simulink model "gm_parallel_prediction_and_cost_function_6phase"  (R2022a)
settings: Solver=FixedStepDiscrete  StartTime=0.0  StopTime=10.0  RelTol=1e-3
undefined symbols (not defined in the file or in its folder): f_c, L_d, L_q, L_x, L_y, p, psi_pm, R_ph
libraries: hdlmdlgenlib x2
(part 1 of 8)
settings Model: Creator=Andre Merx  LastModifiedBy=Andre Merx
settings SolverCC: AlgebraicLoopSolver=TrustRegion
settings DataIOCC: LimitDataPoints=on  SaveOutput=off  SaveTime=off
settings OptimizationCC: BlockReduction=off  ConditionallyExecuteInputs=off  DefaultParameterBehavior=Inlined  LifeSpan=inf
settings DebuggingCC: AlgebraicLoopMsg=error  InheritedTsInSrcMsg=none  SingleTaskRateTransMsg=error  UnconnectedInputMsg=warning  UnconnectedOutputMsg=warning  UnconnectedLineMsg=warning  AllowSymbolicDim=off  StrictBusMsg=ErrorOnBusTreatedAsVector  SFUnexpectedBacktrackingDiag=warning  SFNoUnconditionalDefaultTransitionDiag=warning  SFExecutionAtInitializationDiag=none  SFMachineParentedDataDiag=warning  ArithmeticOperatorsInVariantConditions=warning
settings HardwareCC: ProdBitPerPointer=32  ProdBitPerSizeT=32  ProdBitPerPtrDiffT=32  ProdLargestAtomicFloat=None  ProdIntDivRoundTo=Undefined  ProdEndianess=Unspecified  ProdWordSize=32  ProdHWDeviceType=ASIC/FPGA->ASIC/FPGA  ProdEqTarget=off
settings SFSimCC: SimUseLocalCustomCode=off  CustomCodeUndefinedFunction=UseInterfaceOnly
settings RTWCC: RTWUseLocalCustomCode=off
settings CodeAppCC: StateflowObjectComments=on
settings GRTTargetCC: TargetLangStandard=C89/C90 (ANSI)
settings ConfigComp: CovScope=ReferencedModels  CovMetricSettings=dw  CovSaveCumulativeToWorkspaceVar=on  CovSaveSingleToWorkspaceVar=on  CovExternalEMLEnable=off  CovSFcnEnable=off

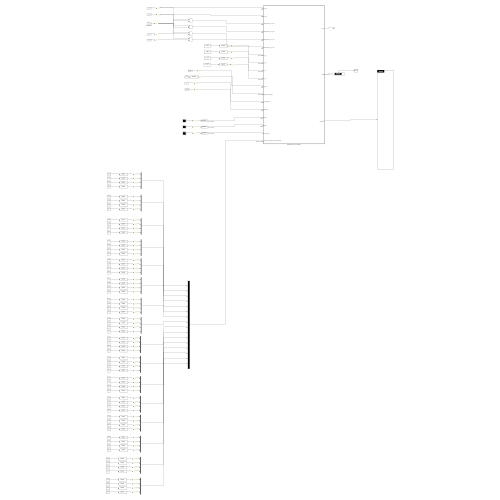
[thumbnail: Simulink's stored preview of the top-level diagram]
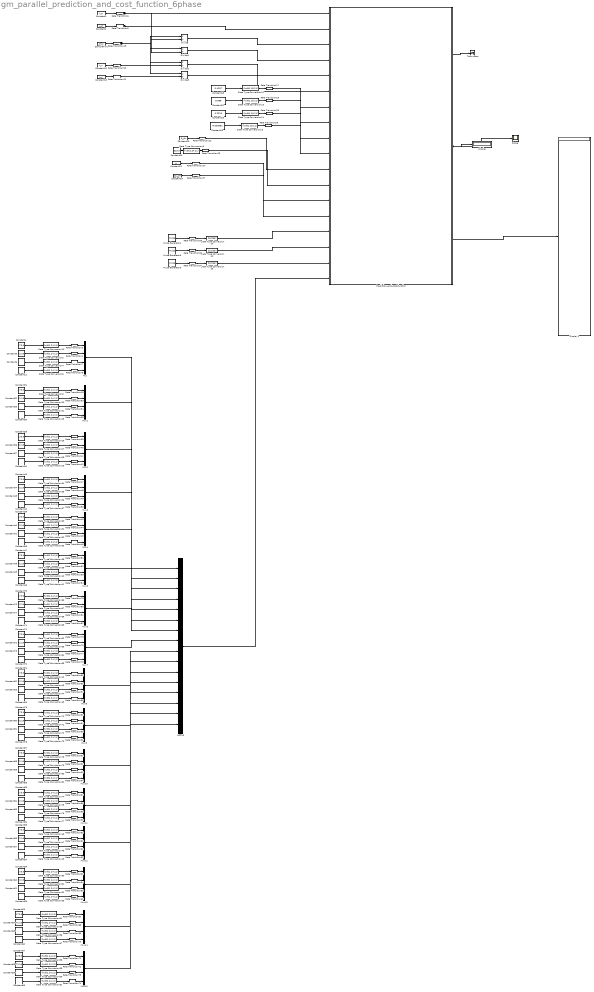
== system gm_parallel_prediction_and_cost_function_6phase ==
  Constant1 : Constant  Value=L_d  OutDataTypeStr=single  SampleTime=-1
  Constant{11,30,34,38,42,46,50,54,58,62,66,70,74,78,82,86} (16 alike) : Constant  Value=-163.1
  Constant12 : Constant  Value=L_x  OutDataTypeStr=single  SampleTime=-1
  Constant13 : Constant  Value=L_y  OutDataTypeStr=single  SampleTime=-1
  Constant18 : Constant  Value=0.4297
  Constant19 : Constant  Value=R_ph  OutDataTypeStr=single  SampleTime=-1
  Constant2 : Constant  Value=L_q  OutDataTypeStr=single  SampleTime=-1
  Constant20 : Constant  Value=313.3
  Constant21 : Constant  Value=p  OutDataTypeStr=single  SampleTime=-1
  Constant22 : Constant  Value=9.988
  Constant23 : Constant  Value=0.2219
  Constant24 : Constant  Value=psi_pm  OutDataTypeStr=single  SampleTime=-1
  Constant25 : Constant  Value=-0.003051
  Constant{4,31,35,39,43,47,51,55,59,63,67,71,75,79,83,87} (16 alike) : Constant  Value=173.9
  Constant{5,32,36,40,44,48,52,56,60,64,68,72,76,80,84,88} (16 alike) : Constant  Value=72.19
  Constant{6,33,37,41,45,49,53,57,61,65,69,73,77,81,85,89} (16 alike) : Constant  Value=-94.17
  Data Type Conversion{2..6,10,20..21,25..81} (65 alike) : DataTypeConversion  OutDataTypeStr=fixdt(1,24,11)  SaturateOnIntegerOverflow=off  RndMeth=Floor
  Data Type Conversion{12..15} (4 alike) : DataTypeConversion  OutDataTypeStr=fixdt(1,18,11)  SaturateOnIntegerOverflow=off  RndMeth=Floor
  Data Type Conversion22 : DataTypeConversion  OutDataTypeStr=boolean  SaturateOnIntegerOverflow=off  RndMeth=Floor
  Data Type Conversion23 : DataTypeConversion  OutDataTypeStr=boolean  SaturateOnIntegerOverflow=off  RndMeth=Floor
  Data Type Conversion24 : DataTypeConversion  OutDataTypeStr=boolean  SaturateOnIntegerOverflow=off  RndMeth=Floor
  Display : Display
  Display1 : Display
  Divide{,1..3} (4 alike) : Product  Inputs=*/  RndMeth=Zero  SaturateOnIntegerOverflow=on
  Mux{,1..15} (16 alike) : Mux
  Mux16 : Mux  Inputs=16
  Prediction_and_cost_function : Subsystem  TreatAsAtomicUnit=on
  Pulse Generator4 : DiscretePulseGenerator  PulseType=Time based  Period=1/f_c
  Pulse Generator5 : DiscretePulseGenerator  PulseType=Time based  Period=1/f_c
  Pulse Generator6 : DiscretePulseGenerator  PulseType=Time based  Period=1/f_c
  Rate Transition{3..8,17..28,33..94} (80 alike) : RateTransition  OutPortSampleTime=Rt
  SampleTime : Constant  Value=1/f_c  OutDataTypeStr=single  SampleTime=-1
  Scope : Scope
  Terminator : Terminator
  wires:
  Prediction_and_cost_function/3(Prediction) -> Display1/1
  Prediction_and_cost_function/1(done) -> Terminator/1
  Prediction_and_cost_function/2(Index) -> Display/1, Scope/1
  Mux16/1 -> Prediction_and_cost_function/18(dqxy_phase_voltage_per_switching_state)
  Mux15/1 -> Mux16/16
  Mux14/1 -> Mux16/15
  Mux13/1 -> Mux16/14
  Mux12/1 -> Mux16/13
  Mux11/1 -> Mux16/12
  Mux10/1 -> Mux16/11
  Mux9/1 -> Mux16/10
  Mux8/1 -> Mux16/9
  Mux7/1 -> Mux16/8
  Mux6/1 -> Mux16/7
  Mux5/1 -> Mux16/6
  Mux4/1 -> Mux16/5
  Mux3/1 -> Mux16/4
  Mux2/1 -> Mux16/3
  Mux1/1 -> Mux16/2
  Mux/1 -> Mux16/1
  Rate Transition74/1 -> Mux15/4
  Rate Transition73/1 -> Mux15/3
  Rate Transition72/1 -> Mux15/2
  Rate Transition71/1 -> Mux15/1
  Rate Transition70/1 -> Mux14/4
  Rate Transition69/1 -> Mux14/3
  Rate Transition68/1 -> Mux14/2
  Rate Transition67/1 -> Mux14/1
  Rate Transition66/1 -> Mux13/4
  Rate Transition65/1 -> Mux13/3
  Rate Transition64/1 -> Mux13/2
  Rate Transition63/1 -> Mux13/1
  Rate Transition62/1 -> Mux12/4
  Rate Transition61/1 -> Mux12/3
  Rate Transition60/1 -> Mux12/2
  Rate Transition59/1 -> Mux12/1
  Rate Transition90/1 -> Mux11/4
  Rate Transition89/1 -> Mux11/3
  Rate Transition88/1 -> Mux11/2
  Rate Transition87/1 -> Mux11/1
  Rate Transition94/1 -> Mux10/4
  Rate Transition93/1 -> Mux10/3
  Rate Transition92/1 -> Mux10/2
  Rate Transition91/1 -> Mux10/1
  Rate Transition86/1 -> Mux9/4
  Rate Transition85/1 -> Mux9/3
  Rate Transition84/1 -> Mux9/2
  Rate Transition83/1 -> Mux9/1
  Rate Transition57/1 -> Mux8/3
  Rate Transition58/1 -> Mux8/4
  Rate Transition56/1 -> Mux8/2
  Rate Transition55/1 -> Mux8/1
  Rate Transition77/1 -> Mux7/3
  Rate Transition78/1 -> Mux7/4
  Rate Transition76/1 -> Mux7/2
  Rate Transition75/1 -> Mux7/1
  Rate Transition82/1 -> Mux6/4
  Rate Transition81/1 -> Mux6/3
  Rate Transition80/1 -> Mux6/2
  Rate Transition79/1 -> Mux6/1
  Rate Transition54/1 -> Mux5/4
  Rate Transition53/1 -> Mux5/3
  Rate Transition52/1 -> Mux5/2
  Rate Transition51/1 -> Mux5/1
  Rate Transition46/1 -> Mux4/4
  Rate Transition45/1 -> Mux4/3
  Rate Transition44/1 -> Mux4/2
  Rate Transition43/1 -> Mux4/1
  Rate Transition50/1 -> Mux3/4
  Rate Transition49/1 -> Mux3/3
  Rate Transition48/1 -> Mux3/2
  Rate Transition47/1 -> Mux3/1
  Rate Transition42/1 -> Mux2/4
  Rate Transition41/1 -> Mux2/3
  Rate Transition40/1 -> Mux2/2
  Rate Transition39/1 -> Mux2/1
  Rate Transition38/1 -> Mux1/4
  Rate Transition34/1 -> Mux1/3
  Rate Transition33/1 -> Mux1/2
  Rate Transition18/1 -> Mux1/1
  Rate Transition8/1 -> Mux/4
  Rate Transition7/1 -> Mux/3
  Rate Transition4/1 -> Mux/2
  Rate Transition3/1 -> Mux/1
  Data Type Conversion58/1 -> Rate Transition71/1
  Data Type Conversion59/1 -> Rate Transition72/1
  Data Type Conversion60/1 -> Rate Transition73/1
  Constant69/1 -> Data Type Conversion60/1
  Constant66/1 -> Data Type Conversion61/1
  Constant67/1 -> Data Type Conversion58/1
  Constant68/1 -> Data Type Conversion59/1
  Data Type Conversion61/1 -> Rate Transition74/1
  Data Type Conversion54/1 -> Rate Transition67/1
  Data Type Conversion55/1 -> Rate Transition68/1
  Data Type Conversion56/1 -> Rate Transition69/1
  Constant65/1 -> Data Type Conversion56/1
  Constant62/1 -> Data Type Conversion57/1
  Constant63/1 -> Data Type Conversion54/1
  Constant64/1 -> Data Type Conversion55/1
  Data Type Conversion57/1 -> Rate Transition70/1
  Data Type Conversion50/1 -> Rate Transition63/1
  Data Type Conversion51/1 -> Rate Transition64/1
  Data Type Conversion52/1 -> Rate Transition65/1
  Constant61/1 -> Data Type Conversion52/1
  Constant58/1 -> Data Type Conversion53/1
  Constant59/1 -> Data Type Conversion50/1
  Constant60/1 -> Data Type Conversion51/1
  Data Type Conversion53/1 -> Rate Transition66/1
  Data Type Conversion78/1 -> Rate Transition91/1
  Data Type Conversion79/1 -> Rate Transition92/1
  Data Type Conversion80/1 -> Rate Transition93/1
  Constant89/1 -> Data Type Conversion80/1
  Constant86/1 -> Data Type Conversion81/1
  Constant87/1 -> Data Type Conversion78/1
  Constant88/1 -> Data Type Conversion79/1
  Data Type Conversion81/1 -> Rate Transition94/1
  Data Type Conversion74/1 -> Rate Transition87/1
  Data Type Conversion75/1 -> Rate Transition88/1
  Data Type Conversion76/1 -> Rate Transition89/1
  Constant85/1 -> Data Type Conversion76/1
  Constant82/1 -> Data Type Conversion77/1
  Constant83/1 -> Data Type Conversion74/1
  Constant84/1 -> Data Type Conversion75/1
  Data Type Conversion77/1 -> Rate Transition90/1
  Data Type Conversion70/1 -> Rate Transition83/1
  Data Type Conversion71/1 -> Rate Transition84/1
  Data Type Conversion72/1 -> Rate Transition85/1
  Constant81/1 -> Data Type Conversion72/1
  Constant78/1 -> Data Type Conversion73/1
  Constant79/1 -> Data Type Conversion70/1
  Constant80/1 -> Data Type Conversion71/1
  Data Type Conversion73/1 -> Rate Transition86/1
  Data Type Conversion66/1 -> Rate Transition79/1
  Data Type Conversion67/1 -> Rate Transition80/1
  Data Type Conversion68/1 -> Rate Transition81/1
  Constant77/1 -> Data Type Conversion68/1
  Constant74/1 -> Data Type Conversion69/1
  Constant75/1 -> Data Type Conversion66/1
  Constant76/1 -> Data Type Conversion67/1
  Data Type Conversion69/1 -> Rate Transition82/1
  Data Type Conversion62/1 -> Rate Transition75/1
  Data Type Conversion63/1 -> Rate Transition76/1
  Data Type Conversion64/1 -> Rate Transition77/1
  Constant73/1 -> Data Type Conversion64/1
  Constant70/1 -> Data Type Conversion65/1
  Constant71/1 -> Data Type Conversion62/1
  Constant72/1 -> Data Type Conversion63/1
  Data Type Conversion65/1 -> Rate Transition78/1
  Data Type Conversion46/1 -> Rate Transition59/1
  Data Type Conversion47/1 -> Rate Transition60/1
  Data Type Conversion48/1 -> Rate Transition61/1
  Constant57/1 -> Data Type Conversion48/1
  Constant54/1 -> Data Type Conversion49/1
  Constant55/1 -> Data Type Conversion46/1
  Constant56/1 -> Data Type Conversion47/1
  Data Type Conversion49/1 -> Rate Transition62/1
  Data Type Conversion42/1 -> Rate Transition55/1
  Data Type Conversion43/1 -> Rate Transition56/1
  Data Type Conversion44/1 -> Rate Transition57/1
  Constant53/1 -> Data Type Conversion44/1
  Constant50/1 -> Data Type Conversion45/1
  Constant51/1 -> Data Type Conversion42/1
  Constant52/1 -> Data Type Conversion43/1
  Data Type Conversion45/1 -> Rate Transition58/1
  Data Type Conversion38/1 -> Rate Transition51/1
  Data Type Conversion39/1 -> Rate Transition52/1
  Data Type Conversion40/1 -> Rate Transition53/1
  Constant49/1 -> Data Type Conversion40/1
  Constant46/1 -> Data Type Conversion41/1
  Constant47/1 -> Data Type Conversion38/1
  Constant48/1 -> Data Type Conversion39/1
  Data Type Conversion41/1 -> Rate Transition54/1
  Data Type Conversion34/1 -> Rate Transition47/1
  Data Type Conversion35/1 -> Rate Transition48/1
  Data Type Conversion36/1 -> Rate Transition49/1
  Constant45/1 -> Data Type Conversion36/1
  Constant42/1 -> Data Type Conversion37/1
  Constant43/1 -> Data Type Conversion34/1
  Constant44/1 -> Data Type Conversion35/1
  Data Type Conversion37/1 -> Rate Transition50/1
  Data Type Conversion30/1 -> Rate Transition43/1
  Data Type Conversion31/1 -> Rate Transition44/1
  Data Type Conversion32/1 -> Rate Transition45/1
  Constant41/1 -> Data Type Conversion32/1
  Constant38/1 -> Data Type Conversion33/1
  Constant39/1 -> Data Type Conversion30/1
  Constant40/1 -> Data Type Conversion31/1
  Data Type Conversion33/1 -> Rate Transition46/1
  Data Type Conversion26/1 -> Rate Transition39/1
  Data Type Conversion27/1 -> Rate Transition40/1
  Data Type Conversion28/1 -> Rate Transition41/1
  Constant37/1 -> Data Type Conversion28/1
  Constant34/1 -> Data Type Conversion29/1
  Constant35/1 -> Data Type Conversion26/1
  Constant36/1 -> Data Type Conversion27/1
  Data Type Conversion29/1 -> Rate Transition42/1
  Data Type Conversion3/1 -> Rate Transition18/1
  Data Type Conversion20/1 -> Rate Transition33/1
  Data Type Conversion21/1 -> Rate Transition34/1
  Constant33/1 -> Data Type Conversion21/1
  Constant30/1 -> Data Type Conversion25/1
  Constant31/1 -> Data Type Conversion3/1
  Constant32/1 -> Data Type Conversion20/1
  Data Type Conversion25/1 -> Rate Transition38/1
  Pulse Generator4/1 -> Rate Transition35/1
  Data Type Conversion22/1 -> Prediction_and_cost_function/16(Reset)  "curent_valid_in"
  Pulse Generator5/1 -> Rate Transition36/1
  Rate Transition35/1 -> Data Type Conversion24/1
  Data Type Conversion23/1 -> Prediction_and_cost_function/17(valid_in_ADC)  "curent_valid_in"
  Rate Transition36/1 -> Data Type Conversion22/1
  Data Type Conversion24/1 -> Prediction_and_cost_function/15(valid_in)  "curent_valid_in"
  Pulse Generator6/1 -> Rate Transition37/1
  Rate Transition37/1 -> Data Type Conversion23/1
  Rate Transition27/1 -> Prediction_and_cost_function/14(psiPM_AXI)
  Rate Transition24/1 -> Prediction_and_cost_function/13(pole_pairs_AXI)
  Rate Transition23/1 -> Prediction_and_cost_function/12(omega_m_measured)
  Rate Transition22/1 -> Prediction_and_cost_function/11(Rs_AXI)
  Rate Transition28/1 -> Prediction_and_cost_function/10(iy_k_1)
  Rate Transition17/1 -> Prediction_and_cost_function/7(id_k_1)
  Data Type Conversion12/1 -> Rate Transition17/1
  Constant24/1 -> Rate Transition27/1
  Data Type Conversion15/1 -> Rate Transition28/1
  Rate Transition6/1 -> Prediction_and_cost_function/1(Lq_AXI), Divide1/2
  Data Type Conversion4/1 -> Rate Transition7/1
  Constant22/1 -> Data Type Conversion13/1
  Constant6/1 -> Data Type Conversion4/1
  Data Type Conversion14/1 -> Rate Transition26/1
  Rate Transition26/1 -> Prediction_and_cost_function/9(ix_k_1)
  Rate Transition5/1 -> Prediction_and_cost_function/2(Ld_AXI), Divide/2
  Data Type Conversion2/1 -> Rate Transition4/1
  Divide3/1 -> Prediction_and_cost_function/6(SampleTime_div_Ly_AXI)
  Constant18/1 -> Data Type Conversion12/1
  Constant25/1 -> Data Type Conversion15/1
  Constant20/1 -> Data Type Conversion5/1
  Data Type Conversion5/1 -> Rate Transition23/1
  Constant12/1 -> Rate Transition20/1
  Constant21/1 -> Rate Transition24/1
  Constant23/1 -> Data Type Conversion14/1
  Rate Transition25/1 -> Prediction_and_cost_function/8(iq_k_1)
  Constant19/1 -> Rate Transition22/1
  Constant11/1 -> Data Type Conversion6/1
  Constant2/1 -> Rate Transition6/1
  Constant5/1 -> Data Type Conversion2/1
  Constant4/1 -> Data Type Conversion10/1
  Data Type Conversion13/1 -> Rate Transition25/1
  Constant13/1 -> Rate Transition21/1
  Divide/1 -> Prediction_and_cost_function/3(SampleTime_div_Ld_AXI)
  Data Type Conversion10/1 -> Rate Transition3/1
  Data Type Conversion6/1 -> Rate Transition8/1
  Divide2/1 -> Prediction_and_cost_function/5(SampleTime_div_Lx_AXI)
  Constant1/1 -> Rate Transition5/1
  Rate Transition21/1 -> Divide3/2
  Rate Transition19/1 -> Divide/1, Divide2/1, Divide3/1, Divide1/1
  Rate Transition20/1 -> Divide2/2
  SampleTime/1 -> Rate Transition19/1
  Divide1/1 -> Prediction_and_cost_function/4(SampleTime_div_Lq_AXI)
